simulink model "_autosave_check"  (R2025a)
settings: Solver=FixedStepDiscrete  StartTime=0.0  StopTime=10  FixedStep=0.01  RelTol=1e-3
(part 2 of 2)

== stateflow chart _autosave_check/MainSubsystem/LRM_MLR_ManageLaneRole/MLR_STM_Chart ==
  state MLR_STM_Init
    en: u8LaneRole = uint8(1);
  state MLR_STM_Disabled
    en: u8LaneRole = uint8(5);
  state MLR_STM_ShuttingDown
    en: u8LaneRole = uint8(6);
  state MLR_STM_OperationalRoles
  state MLR_STM_FallBack
    en: u8LaneRole = uint8(3);
  state MLR_STM_Support
    en: u8LaneRole = uint8(4);
  state MLR_STM_Master
    en: u8LaneRole = uint8(2);
  (default) -> MLR_STM_Init [order 1]
  MLR_STM_ShuttingDown -> MLR_STM_Init : [bNotShutdown]
  MLR_STM_Init -> MLR_STM_Disabled [order 2] : [bLclDisabled]
  (default) -> MLR_STM_FallBack [order 2]
  MLR_STM_Disabled -> MLR_STM_ShuttingDown : [bShutdown]
  MLR_STM_OperationalRoles -> MLR_STM_ShuttingDown [order 1] : [bShutdown]
  MLR_STM_Init -> MLR_STM_ShuttingDown [order 1] : [bShutdown]
  MLR_STM_Init -> MLR_STM_FallBack [order 4] : [bArbRmtMaster]
  MLR_STM_Init -> MLR_STM_Master [order 3] : [bArbLclGtRmt]
  MLR_STM_OperationalRoles -> MLR_STM_Disabled [order 2] : [bLclDisabled]
  MLR_STM_FallBack -> MLR_STM_Master [order 1] : [bFallback2Master]
  MLR_STM_Master -> MLR_STM_FallBack [order 2] : [bMaster2Fallback]
  MLR_STM_FallBack -> MLR_STM_Support [order 3] : [bFallback2Support]
  MLR_STM_FallBack -> MLR_STM_Support [order 4] : [bFallback2SupportUnknown]
  MLR_STM_Support -> MLR_STM_FallBack [order 3] : [bSupport2Fallback]
  MLR_STM_FallBack -> MLR_STM_Master [order 2] : [bFallback2MasterTakeover]
  MLR_STM_Master -> MLR_STM_FallBack [order 3] : [bMaster2FallbackImmediate]
  MLR_STM_Support -> MLR_STM_Master [order 2] : [bSupport2MasterTakeover]
  MLR_STM_Support -> MLR_STM_Master [order 1] : [bSupport2Master]
  MLR_STM_Master -> MLR_STM_Support [order 1] : [bMaster2Support]
  data: bShutdown input boolean; bNotShutdown input boolean; bLclDisabled input boolean; bArbLclGtRmt input boolean; bArbRmtMaster input boolean; bMaster2Support input boolean; bMaster2Fallback input boolean; bMaster2FallbackImmediate input boolean; bFallback2Master input boolean; bFallback2MasterTakeover input boolean; bFallback2Support input boolean; bFallback2SupportUnknown input boolean; bSupport2Master input boolean; bSupport2MasterTakeover input boolean; bSupport2Fallback input boolean; u8LaneRole output uint8 size=1

== stateflow chart _autosave_check/MainSubsystem/LRM_MLS_ManageLaneStatus/MLS_STM_StateMachine/MLS_STM_Chart ==
  state INIT
    state Failed
      en: u8LaneStatus = uint8(3);
      en: bMonActive = false;
  state Operating
    en: u8LaneStatus = uint8(1);
    en: bMonActive = true;
  state HbLost
    en: u8LaneStatus = uint8(2);
    en: bMonActive = false;
  state MonitoringOff
    en: u8LaneStatus = uint8(0);
    en: bMonActive = false;
  state MonitoringOn
    en: u8LaneStatus = uint8(0);
    en: bMonActive = true;
  (default) -> INIT [order 1]
  Failed -> HbLost [order 2] : [bIlcFull]
  Failed -> Operating [order 1] : [bHbOk]
  Operating -> Failed [order 1] : [bFailedCond]
  MonitoringOn -> Operating [order 1] : [bHlthOk]
  HbLost -> Operating : [bHbOk]
  Operating -> HbLost [order 2] : [bHbLostCond]
  MonitoringOn -> Failed [order 2] : [bFailedCond]
  MonitoringOn -> HbLost [order 3] : [bHbLostCond]
  (default) -> MonitoringOff [order 2]
  MonitoringOff -> MonitoringOn : [bMonitoringActive]
  data: bMonitoringActive input boolean; bHlthOk input boolean; bHbOk input boolean; bIlcFull input boolean; bHbLostCond input boolean; bFailedCond input boolean; u8LaneStatus output uint8 size=1; bMonActive output boolean size=1
